simulink model "filter_bypass_feedback"  (R2015b)
settings: Solver=VariableStepAuto  StartTime=0.0  StopTime=100.0  RelTol=1e-3
settings Model: Creator=dell  LastModifiedBy=dell

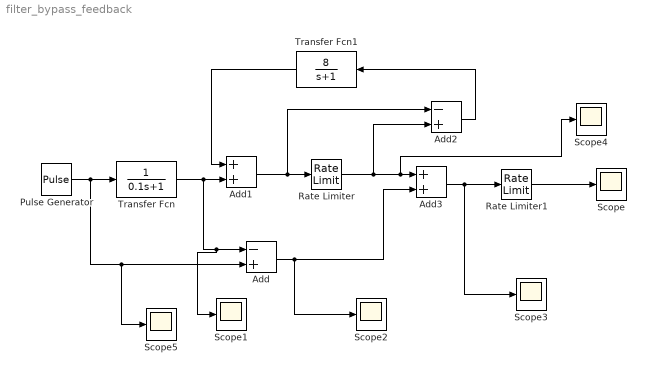
== system filter_bypass_feedback ==
  Add : Sum  Inputs=-+
  Add1 : Sum
  Add2 : Sum  Inputs=-+
  Add3 : Sum
  Pulse Generator : DiscretePulseGenerator  PulseType=Time based  Period=10  PulseWidth=40
  Rate Limiter : RateLimiter  SampleTimeMode=inherited
  Rate Limiter1 : RateLimiter  SampleTimeMode=inherited
  Scope{,1..5} (6 alike) : Scope
  Transfer Fcn : TransferFcn  Denominator=[0.1 1]
  Transfer Fcn1 : TransferFcn  Numerator=[8]  Denominator=[1 1]
  wires:
  Pulse Generator/1 -> Scope5/1, Add/2, Transfer Fcn/1
  Transfer Fcn/1 -> Scope1/1, Add/1, Add1/2
  Add1/1 -> Add2/1, Rate Limiter/1
  Rate Limiter/1 -> Add2/2, Scope4/1, Add3/1
  Add/1 -> Scope2/1, Add3/2
  Add3/1 -> Scope3/1, Rate Limiter1/1
  Add2/1 -> Transfer Fcn1/1
  Transfer Fcn1/1 -> Add1/1
  Rate Limiter1/1 -> Scope/1
